simulink model "flushing_queue_with_priority"  (Simulink 7.4)
settings: Solver=ode45  StartTime=0.0  StopTime=20.0  MaxStep=inf  RelTol=1e-3
undefined symbols (not defined in the file): des_subsystemblock, des_subsysteminport, des_subsystemoutport, des_subsystemsupportblock
libraries: simeventssink1 x6, simeventsrouting1 x4, simulink x2, simeventsattributes2 x2, simeventstranslate1 x2, simeventsqueue1 x2, simeventsgates1 x1, simeventsserver1 x1, simeventsgenerators1 x1
settings Model: Creator=The MathWorks Inc.  LastModifiedBy=wagner  ExtModeAutoUpdateStatusClock=off
settings DataIOCC: SaveOutput=off  SignalLogging=off  SaveTime=off
settings OptimizationCC: InitFltsAndDblsToZero=on
settings DebuggingCC: AlgebraicLoopMsg=error  SolverPrmCheckMsg=none
settings GRTTargetCC: TargetFcnLib=ansi_tfl_tmw_new.mat
settings SimEventsCC: propDiagAttribOutput=1  propDiagFcnCallOutput=1  propDiagStatOutput=0

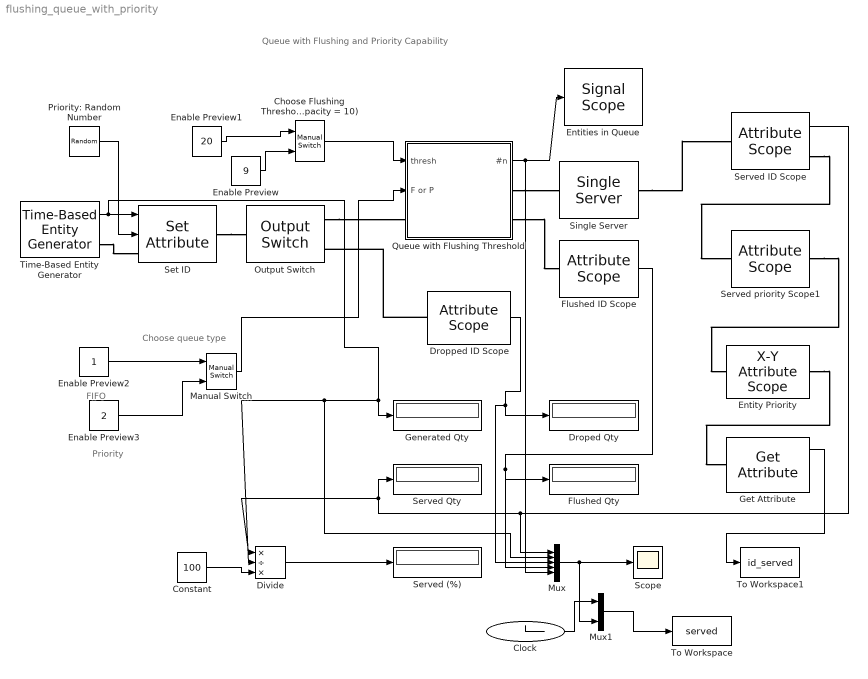
== system flushing_queue_with_priority ==
  note: Queue with Flushing and Priority Capability
  note: Choose queue type
  note: FIFO
  note: Priority
  Choose Flushing Threshold (queue capacity = 10) : simulink/Signal Routing/Manual Switch  SystemSampleTime=-1  sw=0  action=0  varsize=off
  Clock : Clock
      settings: Decimation=10
  Constant : Constant  Value=100  OutDataType=fixdt(1, 16)  OutScaling=2^0
  Divide : Product  Inputs=*/*  OutDataType=fixdt(1, 16)  OutScaling=2^-10
  Droped Qty : Display
  Dropped ID Scope : simeventssink1/Attribute Scope  Priority=1  SystemSampleTime=-1  PlotType=Stair  InputType=Attribute  NumInputs=1  AttributeNameY=ID  XInputOptionSignal=Event time  XInputOptionEntity=Event time  AttributeNameX=Count  EnableEntityOutport=off  XMin=0  XMax=10  XLimitExceededOption=Stretch axis limits  YLimitExceededOption=Stretch axis limits  AxisGrid=on  AxisLegend=off  LineDisables=""  LineColors=b  LineStyles=None  LineMarkers=.  OpenScopeAtSimStart=on  Title=ID of Dropped Entities  YLabel=ID  XLabel=Time  FigurePosition=[7 505 480 272]  AxisZoom=off  DataStoreOption=Limited  DataPointsLimit=10000  StatNumberArrived=On  ShowCountPlotted=on  ShowToolbar=off
      settings: YMin=0  YMax=10
  Enable Preview : Constant  Value=9  OutDataType=sfix(16)  OutScaling=2^0
  Enable Preview1 : Constant  Value=20  OutDataType=sfix(16)  OutScaling=2^0
  Enable Preview2 : Constant  Description=FIFO  OutDataType=sfix(16)  OutScaling=2^0
  Enable Preview3 : Constant  Description=FIFO  Value=2  OutDataType=sfix(16)  OutScaling=2^0
  Entities in Queue : simeventssink1/Signal Scope  Priority=1  SystemSampleTime=-1  PlotType=Stair  InputType=Signal  NumInputs=1  AttributeNameY=Count  XInputOptionSignal=Event time  XInputOptionEntity=Event time  AttributeNameX=Count  EnableEntityOutport=on  XMin=0  XMax=10  XLimitExceededOption=Stretch axis limits  YLimitExceededOption=Stretch axis limits  AxisGrid=on  AxisLegend=off  LineDisables=""  LineColors="1  0  0"  LineStyles=-  LineMarkers=.  OpenScopeAtSimStart=on  Title=Entities in Queue  YLabel=Entities  XLabel=Time  FigurePosition=[7 505 480 272]  AxisZoom=off  DataStoreOption=Limited  DataPointsLimit=10000  StatNumberArrived=Off  ShowCountPlotted=off  ShowToolbar=off
      settings: YMin=0  YMax=10
  Entity Priority : simeventssink1/X-Y Attribute Scope  Priority=1  SystemSampleTime=-1  PlotType=Continuous  InputType=Attribute  NumInputs=1  AttributeNameY=priority  XInputOptionSignal=Event time  XInputOptionEntity=Attribute  AttributeNameX=ID  EnableEntityOutport=on  XMin=0  XMax=50  XLimitExceededOption=Stretch axis limits  YLimitExceededOption=Stretch axis limits  AxisGrid=on  AxisLegend=off  LineDisables=""  LineColors=b  LineStyles=-  LineMarkers=diamond  OpenScopeAtSimStart=on  Title=Priority of entities (with path): The lower the number the more priority that entity gets  YLabel=Priority  XLabel=ID  FigurePosition=[7 505 480 272]  AxisZoom=off  DataStoreOption=Limited  DataPointsLimit=10000  StatNumberArrived=Off  ShowCountPlotted=on  ShowToolbar=off
      settings: YMin=-10  YMax=10
  Flushed ID Scope : simeventssink1/Attribute Scope  Priority=1  SystemSampleTime=-1  PlotType=Stair  InputType=Attribute  NumInputs=1  AttributeNameY=ID  XInputOptionSignal=Event time  XInputOptionEntity=Event time  AttributeNameX=Count  EnableEntityOutport=off  XMin=0  XMax=10  XLimitExceededOption=Stretch axis limits  YLimitExceededOption=Stretch axis limits  AxisGrid=on  AxisLegend=off  LineDisables=""  LineColors=b  LineStyles=None  LineMarkers=.  OpenScopeAtSimStart=on  Title=ID of Flushed Entities  YLabel=ID  XLabel=Time  FigurePosition=[7 505 480 272]  AxisZoom=off  DataStoreOption=Limited  DataPointsLimit=10000  StatNumberArrived=On  ShowCountPlotted=on  ShowToolbar=off
      settings: YMin=0  YMax=10
  Flushed Qty : Display
  Generated Qty : Display
  Get Attribute : simeventsattributes2/Get Attribute  Priority=1  DialogController=des_ddg_create  DialogControllerArgs=DataTag5  SystemSampleTime=-1  AttributeName=ID  AttributeMissing=Default value  AttributeDefaultValue=1  AttributeSendTiming=After entity departure  AttributeTreatAsVector=0  StatNumberDeparted=Off  EvaluatedDefaultAttributeValue={1}
  Manual Switch : simulink/Signal Routing/Manual Switch  SystemSampleTime=-1  sw=0  action=0  varsize=off
  Mux : Mux  Inputs=5
      settings: DisplayOption=signals
  Mux1 : Mux  Inputs=2
  Output Switch : simeventsrouting1/Output Switch  Priority=1  SystemSampleTime=-1  NumberOutputPorts=2  SwitchingCriterion=First port that is not blocked  InitialSeed=34567  AttributeName=Attribute1  InitialConditionsOpt=off  InitialConditions=1  EntityBufferOpt=off  SpecifyEventPriority=off  PriorityOutputSwitchSelectPort=4100  TimeoutPortOpt=off  StatNumberDeparted=Off  StatNumberTimedOut=Off  StatPendingEntity=Off  StatLastDeparturePort=Off  EvaluatedNumPorts=2
  Priority: Random Number : RandomNumber  Variance=10  SampleTime=0.1
  Queue with Flushing Threshold : Subsystem
  Scope : Scope
      settings: TimeRange=20  YMin=0  YMax=140
  Served (%) : Display
  Served ID Scope : simeventssink1/Attribute Scope  Priority=1  SystemSampleTime=-1  PlotType=Stair  InputType=Attribute  NumInputs=1  AttributeNameY=ID  XInputOptionSignal=Event time  XInputOptionEntity=Event time  AttributeNameX=Count  EnableEntityOutport=on  XMin=0  XMax=10  XLimitExceededOption=Stretch axis limits  YLimitExceededOption=Stretch axis limits  AxisGrid=on  AxisLegend=off  LineDisables=""  LineColors=b  LineStyles=None  LineMarkers=.  OpenScopeAtSimStart=on  Title=ID of Served Entities  YLabel=ID  XLabel=Time  FigurePosition=[7 505 480 272]  AxisZoom=off  DataStoreOption=Limited  DataPointsLimit=10000  StatNumberArrived=On  ShowCountPlotted=on  ShowToolbar=off
      settings: YMin=0  YMax=10
  Served Qty : Display
  Served priority Scope1 : simeventssink1/Attribute Scope  Priority=1  SystemSampleTime=-1  PlotType=Stair  InputType=Attribute  NumInputs=1  AttributeNameY=priority  XInputOptionSignal=Event time  XInputOptionEntity=Event time  AttributeNameX=Count  EnableEntityOutport=on  XMin=0  XMax=10  XLimitExceededOption=Stretch axis limits  YLimitExceededOption=Stretch axis limits  AxisGrid=on  AxisLegend=off  LineDisables=""  LineColors=b  LineStyles=None  LineMarkers=.  OpenScopeAtSimStart=on  Title=Priority of Served Entities  YLabel=priority  XLabel=Time  FigurePosition=[7 505 480 272]  AxisZoom=off  DataStoreOption=Limited  DataPointsLimit=10000  StatNumberArrived=Off  ShowCountPlotted=on  ShowToolbar=off
      settings: YMin=0  YMax=10
  Set ID : simeventsattributes2/Set Attribute  Priority=1  DialogController=des_ddg_create  DialogControllerArgs=DataTag25  SystemSampleTime=-1  AttributeFrom=Signal port|Signal port  AttributeName=ID|priority  AttributeTreatAsVector=1|1  AttributeValue=1|1  AttributeCreate=on  StatNumberDeparted=Off  EvaluatedAttributeValue={[];[]}
  Single Server : simeventsserver1/Single Server  Priority=1  SystemSampleTime=-1  ServiceTimeFrom=Dialog  ServiceTime=.27  AttributeName=ServiceTime  PriorityServiceCompletion=500  PermitPreemption=off  SortingAttributeName=PriorityAttributeName  SortingDirection=Ascending  WriteToAttribute=off  ResidualAttributeName=ResidualServiceTime  CreateAttribute=on  EnableTOPort=off  StatNumberDeparted=Off  StatNumberInBlock=Off  StatNumberPreempted=Off  StatPendingEntity=Off  StatAverageWait=Off  StatUtilization=Off  StatNumberTimedout=Off
  Time-Based Entity Generator : simeventsgenerators1/Entity Generators/Time-Based Entity Generator  Priority=1  DialogController=des_ddg_create  DialogControllerArgs=DataTag28  SystemSampleTime=-1  GenerateEntitiesUpon=Intergeneration time from dialog  Distribution=Exponential  Minimum=0  Maximum=.7  Mean=.15  InitialSeed=12345  Period=.3  PriorityEntityGeneration=600  GenerateEntityAtSimulationStart=off  ResponseWhenBlocked=Error  ResponseWhenUnblocked=Immediate restart  EntityType=Blank  StatNumberDeparted=On  StatPendingEntity=Off  StatAverageIntergenerationTime=Off
  To Workspace : ToWorkspace  VariableName=served  SampleTime=-1  SaveFormat=Array
  To Workspace1 : ToWorkspace  VariableName=id_served  SampleTime=-1  SaveFormat=Array
  wires:
  Choose Flushing Threshold (queue capacity = 10)/1 -> Queue with Flushing Threshold/1(thresh)
  Queue with Flushing Threshold/1(#n) -> Entities in Queue/1, Mux/5
  Time-Based Entity Generator/1 -> Set ID/1, Generated Qty/1, Divide/2, Mux/2
  Enable Preview1/1 -> Choose Flushing Threshold (queue capacity = 10)/1
  Enable Preview/1 -> Choose Flushing Threshold (queue capacity = 10)/2
  Priority: Random Number/1 -> Set ID/2
  Enable Preview3/1 -> Manual Switch/2
  Enable Preview2/1 -> Manual Switch/1
  Manual Switch/1 -> Queue with Flushing Threshold/2(F or P)
  Dropped ID Scope/1 -> Droped Qty/1, Mux/3
  Flushed ID Scope/1 -> Flushed Qty/1, Mux/4
  Served ID Scope/1 -> Served Qty/1, Divide/1, Mux/1
  Divide/1 -> Served (%)/1
  Constant/1 -> Divide/3
  Mux/1 -> Scope/1, Mux1/2
  Clock/1 -> Mux1/1
  Mux1/1 -> To Workspace/1
  Get Attribute/1 -> To Workspace1/1
  connections:
  Queue with Flushing Threshold/RConn1 -- Single Server/LConn1
  Time-Based Entity Generator/RConn1 -- Set ID/LConn1
  Queue with Flushing Threshold/RConn2 -- Flushed ID Scope/LConn1
  Set ID/RConn1 -- Output Switch/LConn1
  Output Switch/RConn1 -- Queue with Flushing Threshold/LConn1
  Dropped ID Scope/LConn1 -- Output Switch/RConn2
  Served ID Scope/RConn1 -- Served priority Scope1/LConn1
  Served priority Scope1/RConn1 -- Entity Priority/LConn1
  Single Server/RConn1 -- Served ID Scope/LConn1
  Entity Priority/RConn1 -- Get Attribute/LConn1

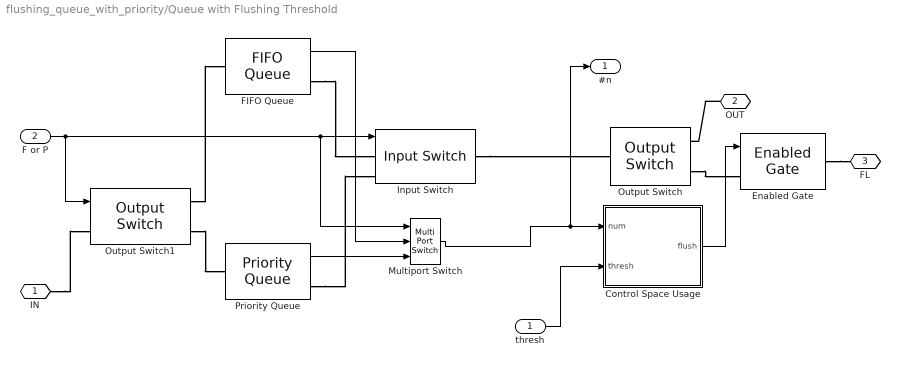
== system flushing_queue_with_priority/Queue with Flushing Threshold ==
  thresh : Inport  OutDataType=sfix(16)  OutScaling=2^0
  F or P : Inport  Port=2  OutDataType=fixdt(1, 16)  OutScaling=2^0
  Control Space Usage : Subsystem  LoadFcn=des_subsystemblock(gcb, 'load');  InitFcn=des_subsystemblock(gcb, 'init');  StartFcn=des_subsystemblock(gcb, 'start');  StopFcn=des_subsystemblock(gcb, 'stop');
      settings: CopyFcn=des_subsystemblock(gcb, 'copy');  DeleteFcn=des_subsystemblock(gcb, 'delete');  UndoDeleteFcn=des_subsystemblock(gcb, 'undodelete');  ModelCloseFcn=des_subsystemblock(gcb, 'modelclose');  PreSaveFcn=des_subsystemblock(gcb, 'presave');  NameChangeFcn=des_subsystemblock(gcb, 'namechange');  OpenFcn=des_subsystemblock(gcb, 'open');  ParentCloseFcn=des_subsystemblock(gcb, 'parentclose');  ErrorFcn=des_subsystemerror
      mask Type: Discrete Event Subsystem
      mask Help: helpview(simeventsbhelp);
  Enabled Gate : simeventsgates1/Enabled Gate  Priority=1  SystemSampleTime=-1  SpecifyEventPriority=off  PriorityGateEnableOpenClose=30  StatNumberDeparted=Off
  FIFO Queue : simeventsqueue1/FIFO Queue  Priority=1  SystemSampleTime=-1  Capacity=10  EnableTOPort=off  StatNumberDeparted=Off  StatNumberInBlock=On  StatPendingEntity=Off  StatAverageWait=Off  StatAverageQueueLength=Off  StatNumberTimedout=Off
      settings: AttributesFormatString=Capacity = %<Capacity>
  Input Switch : simeventsrouting1/Input Switch  Priority=1  SystemSampleTime=-1  NumberInputPorts=2  SwitchingCriterion=From signal port p  InitialSeed=23453  SpecifyEventPriority=off  PriorityInputSwitchSelectPort=4000  StatNumberDeparted=Off  StatLastArrivalPort=Off  EvaluatedNumPorts=2
  Multiport Switch : MultiPortSwitch  Inputs=2  OutDataType=fixdt(1, 16)  OutScaling=2^0
  Output Switch : simeventsrouting1/Output Switch  Priority=1  SystemSampleTime=-1  NumberOutputPorts=2  SwitchingCriterion=First port that is not blocked  InitialSeed=34567  AttributeName=Attribute1  InitialConditionsOpt=off  InitialConditions=1  EntityBufferOpt=off  SpecifyEventPriority=off  PriorityOutputSwitchSelectPort=4100  TimeoutPortOpt=off  StatNumberDeparted=Off  StatNumberTimedOut=Off  StatPendingEntity=Off  StatLastDeparturePort=Off  EvaluatedNumPorts=2
  Output Switch1 : simeventsrouting1/Output Switch  Priority=1  SystemSampleTime=-1  NumberOutputPorts=2  SwitchingCriterion=From signal port p  InitialSeed=34567  AttributeName=Attribute1  InitialConditionsOpt=off  InitialConditions=1  EntityBufferOpt=on  SpecifyEventPriority=off  PriorityOutputSwitchSelectPort=4100  TimeoutPortOpt=off  StatNumberDeparted=Off  StatNumberTimedOut=Off  StatPendingEntity=Off  StatLastDeparturePort=Off  EvaluatedNumPorts=2
  Priority Queue : simeventsqueue1/Priority Queue  Priority=1  SystemSampleTime=-1  Capacity=10  SortingAttributeName=priority  SortingDirection=Ascending  EnableTOPort=off  StatNumberDeparted=Off  StatNumberInBlock=On  StatPendingEntity=Off  StatAverageWait=Off  StatAverageQueueLength=Off  StatNumberTimedout=Off
      settings: AttributesFormatString=Capacidade = %<Capacity>
  IN : PMIOPort  Port=1  Side=Left
  OUT : PMIOPort  Port=2  Side=Right
  FL : PMIOPort  Port=3  Side=Right
  #n : Outport  OutDataType=sfix(16)  OutScaling=2^0
  wires:
  thresh/1 -> Control Space Usage/2(thresh)
  Control Space Usage/1(flush) -> Enabled Gate/1
  F or P/1 -> Output Switch1/1, Input Switch/1, Multiport Switch/1
  FIFO Queue/1 -> Multiport Switch/2
  Priority Queue/1 -> Multiport Switch/3
  Multiport Switch/1 -> #n/1, Control Space Usage/1(num)
  connections:
  Output Switch/RConn2 -- Enabled Gate/LConn1
  OUT/RConn1 -- Output Switch/RConn1
  Enabled Gate/RConn1 -- FL/RConn1
  IN/RConn1 -- Output Switch1/LConn1
  Output Switch1/RConn2 -- Priority Queue/LConn1
  Output Switch1/RConn1 -- FIFO Queue/LConn1
  Priority Queue/RConn1 -- Input Switch/LConn2
  FIFO Queue/RConn1 -- Input Switch/LConn1
  Input Switch/RConn1 -- Output Switch/LConn1

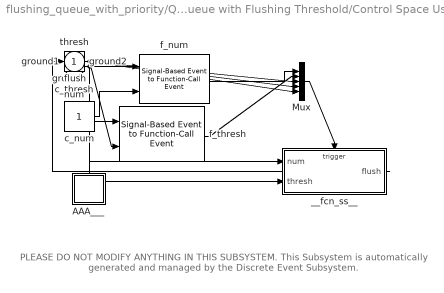
== system flushing_queue_with_priority/Queue with Flushing Threshold/Control Space Usage ==
  note: PLEASE DO NOT MODIFY ANYTHING IN THIS SUBSYSTEM.
      | This Subsystem is automatically generated and
      | managed by the Discrete Event Subsystem.
  num : Inport  DataType=double  OutDataType=sfix(16)  OutScaling=2^0  OutDataTypeStr=double
  thresh : Inport  Port=2  DataType=double  OutDataType=sfix(16)  OutScaling=2^0  OutDataTypeStr=double
  AAA___ : Subsystem  LoadFcn=des_subsystemsupportblock(gcb, 'load');  InitFcn=des_subsystemsupportblock(gcb, 'init');  StartFcn=des_subsystemsupportblock(gcb, 'start');  StopFcn=des_subsystemsupportblock(gcb, 'stop');
      settings: CopyFcn=des_subsystemsupportblock(gcb, 'copy');  DeleteFcn=des_subsystemsupportblock(gcb, 'delete');  UndoDeleteFcn=des_subsystemsupportblock(gcb, 'undodelete');  ModelCloseFcn=des_subsystemsupportblock(gcb, 'modelclose');  PreSaveFcn=des_subsystemsupportblock(gcb, 'presave');  NameChangeFcn=des_subsystemsupportblock(gcb, 'namechange');  OpenFcn=des_subsystemsupportblock(gcb, 'open');  ParentCloseFcn=des_subsystemsupportblock(gcb, 'parentclose');
  Mux : Mux  Inputs=5
  __fcn_ss__ : Subsystem  TreatAsAtomicUnit=on
      settings: PropExecContextOutsideSubsystem=on
  c_num : Constant  OutDataType=sfix(16)  OutScaling=2^0
  c_thresh : Constant  OutDataType=sfix(16)  OutScaling=2^0
  f_num : simeventstranslate1/Signal-Based Event to Function-Call Event  Priority=1  SystemSampleTime=-1  GenerateFunctionCallUpon=Change in signal from port vc  SignalEdgeOption=Either  EnableE1Port=on  EnableF2Port=off  EnableE2Port=off  SpecifyEventPriority=off  PriorityFunctionCall=10  FunctionCallDelayFrom=Dialog  DelayFunctionCall=0  StatNumberF1Calls=Off  StatNumberF2Calls=Off  MaskBlockType=DESS_EVENT_PORT
  f_thresh : simeventstranslate1/Signal-Based Event to Function-Call Event  Priority=1  SystemSampleTime=-1  GenerateFunctionCallUpon=Change in signal from port vc  SignalEdgeOption=Either  EnableE1Port=on  EnableF2Port=off  EnableE2Port=off  SpecifyEventPriority=off  PriorityFunctionCall=20  FunctionCallDelayFrom=Dialog  DelayFunctionCall=0  StatNumberF1Calls=Off  StatNumberF2Calls=Off  MaskBlockType=DESS_EVENT_PORT
  ground : Ground
  ground1 : Ground
  ground2 : Ground
  flush : Outport  OutDataType=sfix(16)  OutScaling=2^0
  wires:
  Mux/1 -> __fcn_ss__/Trigger
  c_num/1 -> f_num/2
  f_num/1 -> Mux/1
  f_thresh/1 -> Mux/2
  c_thresh/1 -> f_thresh/2
  __fcn_ss__/1(flush) -> flush/1
  ground/1 -> Mux/3
  ground1/1 -> Mux/5
  ground2/1 -> Mux/4
  num/1 -> f_num/1, __fcn_ss__/1(num)
  thresh/1 -> f_thresh/1, __fcn_ss__/2(thresh)

== system flushing_queue_with_priority/Queue with Flushing Threshold/Control Space Usage/AAA___ ==

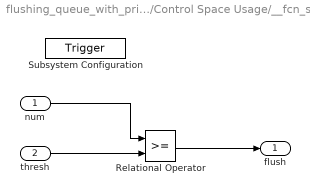
== system flushing_queue_with_priority/Queue with Flushing Threshold/Control Space Usage/__fcn_ss__ ==
  num : Inport  LoadFcn=des_subsysteminport(gcb, 'load');  InitFcn=des_subsysteminport(gcb, 'init');  StartFcn=des_subsysteminport(gcb, 'start');  StopFcn=des_subsysteminport(gcb, 'stop');  OutDataType=sfix(16)  OutScaling=2^0  mask(Discrete Event Inport){PermitSubsystemEvents=on, TypeOfEvent=Change in signal, SignalEdgeOption=Either, SpecifyEventPriority=off, PrioritySubsystemEvent=10}
      mask prompts: PermitSubsystemEvents "Execute subsystem upon signal-based events"; TypeOfEvent "Type of signal-based event:"; SignalEdgeOption "Type of change in signal value:"; SpecifyEventPriority "Resolve simultaneous signal updates according to event priority"; PrioritySubsystemEvent "Event priority:"
      mask help: Input port for a Discrete Event Subsystem block. This block can conditionally execute the subsystem upon signal-based events that meet specified criteria.
      mask init:
      | des_subsystemmask(gcb, 'init','apply')
      settings: CopyFcn=des_subsysteminport(gcb, 'copy');  DeleteFcn=des_subsysteminport(gcb, 'delete');  UndoDeleteFcn=des_subsysteminport(gcb, 'undodelete');  ModelCloseFcn=des_subsysteminport(gcb, 'modelclose');  PreSaveFcn=des_subsysteminport(gcb, 'presave');  NameChangeFcn=des_subsysteminport(gcb, 'namechange');  ParentCloseFcn=des_subsysteminport(gcb, 'parentclose');
      mask Help: helpview(simeventsbhelp);
      mask StyleString: checkbox,popup(Change in signal|Trigger|Sample time hit),popup(Rising|Falling|Either),checkbox,edit
      mask CallbackString: des_subsystemmask(gcb, 'cbPermitSubsystemEvents', 'noapply');|des_subsystemmask(gcb,'cbTypeOfEvent','noapply');||des_subsystemmask(gcb, 'cbSpecifyEventPriority', 'noapply');|
  thresh : Inport  LoadFcn=des_subsysteminport(gcb, 'load');  InitFcn=des_subsysteminport(gcb, 'init');  StartFcn=des_subsysteminport(gcb, 'start');  StopFcn=des_subsysteminport(gcb, 'stop');  Port=2  OutDataType=sfix(16)  OutScaling=2^0  mask(Discrete Event Inport){PermitSubsystemEvents=on, TypeOfEvent=Change in signal, SignalEdgeOption=Either, SpecifyEventPriority=off, PrioritySubsystemEvent=20}
      mask prompts: PermitSubsystemEvents "Execute subsystem upon signal-based events"; TypeOfEvent "Type of signal-based event:"; SignalEdgeOption "Type of change in signal value:"; SpecifyEventPriority "Resolve simultaneous signal updates according to event priority"; PrioritySubsystemEvent "Event priority:"
      mask help: Input port for a Discrete Event Subsystem block. This block can conditionally execute the subsystem upon signal-based events that meet specified criteria.
      mask init:
      | des_subsystemmask(gcb, 'init','apply')
      settings: CopyFcn=des_subsysteminport(gcb, 'copy');  DeleteFcn=des_subsysteminport(gcb, 'delete');  UndoDeleteFcn=des_subsysteminport(gcb, 'undodelete');  ModelCloseFcn=des_subsysteminport(gcb, 'modelclose');  PreSaveFcn=des_subsysteminport(gcb, 'presave');  NameChangeFcn=des_subsysteminport(gcb, 'namechange');  ParentCloseFcn=des_subsysteminport(gcb, 'parentclose');
      mask Help: helpview(simeventsbhelp);
      mask StyleString: checkbox,popup(Change in signal|Trigger|Sample time hit),popup(Rising|Falling|Either),checkbox,edit
      mask CallbackString: des_subsystemmask(gcb, 'cbPermitSubsystemEvents', 'noapply');|des_subsystemmask(gcb,'cbTypeOfEvent','noapply');||des_subsystemmask(gcb, 'cbSpecifyEventPriority', 'noapply');|
  Subsystem Configuration : TriggerPort  TriggerType=function-call
      settings: CopyFcn=des_subsystemconfigblock(gcb, 'copy');  DeleteFcn=des_subsystemconfigblock(gcb, 'delete');  UndoDeleteFcn=des_subsystemconfigblock(gcb, 'undodelete');
      mask Type: Subsystem Configuration
      mask Description: Configuration for a Discrete Event Subsystem block. Every discrete event subsystem window must contain exactly one copy of this configuration block. Do not delete this block.
      mask Help: helpview(simeventsbhelp);
      mask Display: disp('Do Not Delete');
  Relational Operator : RelationalOperator  LogicOutDataTypeMode=Specify via dialog  LogicDataType=float('double')  OutDataTypeStr=float('double')
  flush : Outport  LoadFcn=des_subsystemoutport(gcb, 'load');  InitFcn=des_subsystemoutport(gcb, 'init');  StartFcn=des_subsystemoutport(gcb, 'start');  StopFcn=des_subsystemoutport(gcb, 'stop');  OutDataType=sfix(16)  OutScaling=2^0  mask(Discrete Event Outport){InitOutput=[]}
      mask prompts: InitOutput "Initial output:"
      mask help: Provide an output port for a Discrete Event Subsystem block.
      settings: CopyFcn=des_subsystemoutport(gcb, 'copy');  DeleteFcn=des_subsystemoutport(gcb, 'delete');  UndoDeleteFcn=des_subsystemoutport(gcb, 'undodelete');  ModelCloseFcn=des_subsystemoutport(gcb, 'modelclose');  PreSaveFcn=des_subsystemoutport(gcb, 'presave');  NameChangeFcn=des_subsystemoutport(gcb, 'namechange');  ParentCloseFcn=des_subsystemoutport(gcb, 'parentclose');
      mask Help: helpview(simeventsbhelp);
      mask CallbackString: set_param(gcb,'InitialOutput',get_param(gcb,'InitOutput'));
  wires:
  Relational Operator/1 -> flush/1
  num/1 -> Relational Operator/1
  thresh/1 -> Relational Operator/2
